simulink model "powerwindow01"  (Simulink 6.0)
settings: Solver=ode23  StartTime=0.0  StopTime=inf  FixedStep=1e-4  RelTol=1e-3
libraries: simulink x4
settings Model: Creator=The MathWorks Inc.  LastModifiedBy=batserve  ExtModeAutoUpdateStatusClock=off
settings DataIOCC: SignalLoggingName=sigsOut
settings OptimizationCC: BooleanDataType=off
settings DebuggingCC: CheckExecutionContextPreStartOutputMsg=on  CheckExecutionContextRuntimeOutputMsg=on  SolverPrmCheckMsg=none
settings HardwareCC: TargetUnknown=on

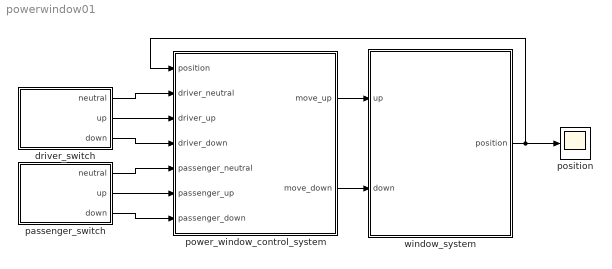
== system powerwindow01 ==
  driver_switch : Subsystem  PropExecContextAcrossSSBoundary=on
  passenger_switch : Subsystem  PropExecContextAcrossSSBoundary=on
  position : Scope
      settings: YMin=-0.05  YMax=0.5  DataFormat=Array
  power_window_control_system : Subsystem  PropExecContextAcrossSSBoundary=on
  window_system : Subsystem  PropExecContextAcrossSSBoundary=on
  wires:
  driver_switch/1(neutral) -> power_window_control_system/2(driver_neutral)
  driver_switch/2(up) -> power_window_control_system/3(driver_up)
  driver_switch/3(down) -> power_window_control_system/4(driver_down)
  passenger_switch/1(neutral) -> power_window_control_system/5(passenger_neutral)
  passenger_switch/2(up) -> power_window_control_system/6(passenger_up)
  passenger_switch/3(down) -> power_window_control_system/7(passenger_down)
  power_window_control_system/1(move_up) -> window_system/1(up)
  power_window_control_system/2(move_down) -> window_system/2(down)
  window_system/1(position) -> position/1, power_window_control_system/1(position)

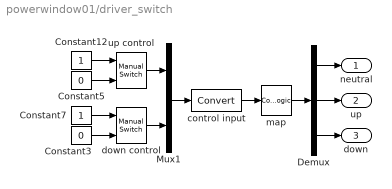
== system powerwindow01/driver_switch ==
  Constant12 : Constant
  Constant3 : Constant  Value=0
  Constant5 : Constant  Value=0
  Constant7 : Constant
  Demux : Demux  Outputs=3
  Mux1 : Mux  Inputs=2
  control input : DataTypeConversion  OutDataTypeMode=boolean  SaturateOnIntegerOverflow=on  RndMeth=Zero
  down control : simulink/Signal Routing/Manual Switch  sw=0  action=0
  map : CombinatorialLogic  TruthTable=[1 0 0;0 0 1;0 1 0;1 0 0]
  up control : simulink/Signal Routing/Manual Switch  sw=0  action=0
  neutral : Outport
  up : Outport  Port=2
  down : Outport  Port=3
  wires:
  control input/1 -> map/1
  Constant12/1 -> up control/1
  Constant5/1 -> up control/2
  Constant7/1 -> down control/1
  Constant3/1 -> down control/2
  down control/1 -> Mux1/2
  Mux1/1 -> control input/1
  up control/1 -> Mux1/1
  map/1 -> Demux/1
  Demux/1 -> neutral/1
  Demux/2 -> up/1
  Demux/3 -> down/1

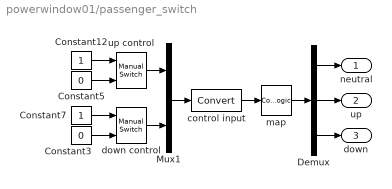
== system powerwindow01/passenger_switch ==
  Constant12 : Constant
  Constant3 : Constant  Value=0
  Constant5 : Constant  Value=0
  Constant7 : Constant
  Demux : Demux  Outputs=3
  Mux1 : Mux  Inputs=2
  control input : DataTypeConversion  OutDataTypeMode=boolean  SaturateOnIntegerOverflow=on  RndMeth=Zero
  down control : simulink/Signal Routing/Manual Switch  sw=0  action=0
  map : CombinatorialLogic  TruthTable=[1 0 0;0 0 1;0 1 0;1 0 0]
  up control : simulink/Signal Routing/Manual Switch  sw=0  action=0
  neutral : Outport
  up : Outport  Port=2
  down : Outport  Port=3
  wires:
  Demux/3 -> down/1
  Demux/2 -> up/1
  Demux/1 -> neutral/1
  map/1 -> Demux/1
  up control/1 -> Mux1/1
  Mux1/1 -> control input/1
  down control/1 -> Mux1/2
  Constant3/1 -> down control/2
  Constant7/1 -> down control/1
  Constant5/1 -> up control/2
  Constant12/1 -> up control/1
  control input/1 -> map/1

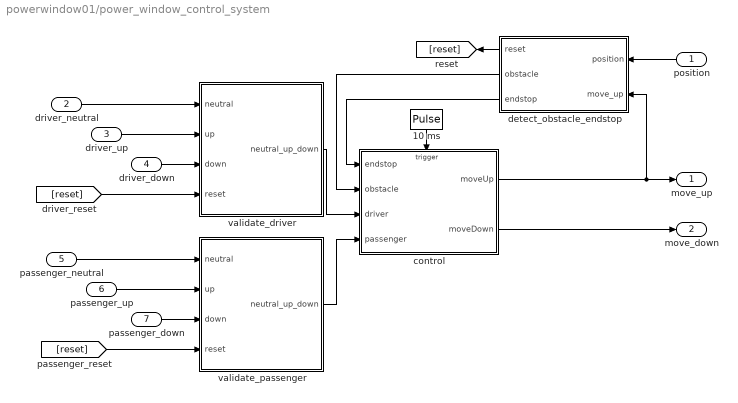
== system powerwindow01/power_window_control_system ==
  position : Inport  Orientation=left  Port=1  LatchInput=off
  driver_neutral : Inport  Port=2  LatchInput=off
  driver_up : Inport  Port=3  LatchInput=off
  driver_down : Inport  Port=4  LatchInput=off
  passenger_neutral : Inport  Port=5  LatchInput=off
  passenger_up : Inport  Port=6  LatchInput=off
  passenger_down : Inport  Port=7  LatchInput=off
  10 ms : DiscretePulseGenerator  Orientation=down  SampleTime=10e-3
  control : Stateflow chart  TreatAsAtomicUnit=on  PropExecContextAcrossSSBoundary=on
  detect_obstacle_endstop : Subsystem  Orientation=left  PropExecContextAcrossSSBoundary=on
  validate_driver : Subsystem  PropExecContextAcrossSSBoundary=on
  validate_passenger : Subsystem  PropExecContextAcrossSSBoundary=on
  move_up : Outport
  move_down : Outport  Port=2
  wires:
  detect_obstacle_endstop/2(obstacle) -> control/2(obstacle)
  detect_obstacle_endstop/3(endstop) -> control/1(endstop)
  detect_obstacle_endstop/1(reset) -> [reset]
  position/1 -> detect_obstacle_endstop/1(position)
  10 ms/1 -> control/Trigger
  control/1(moveUp) -> detect_obstacle_endstop/2(move_up), move_up/1
  control/2(moveDown) -> move_down/1
  driver_neutral/1 -> validate_driver/1(neutral)
  driver_up/1 -> validate_driver/2(up)
  driver_down/1 -> validate_driver/3(down)
  [reset] -> validate_driver/4(reset)
  passenger_neutral/1 -> validate_passenger/1(neutral)
  passenger_up/1 -> validate_passenger/2(up)
  passenger_down/1 -> validate_passenger/3(down)
  [reset] -> validate_passenger/4(reset)
  validate_driver/1(neutral_up_down) -> control/3(driver)
  validate_passenger/1(neutral_up_down) -> control/4(passenger)

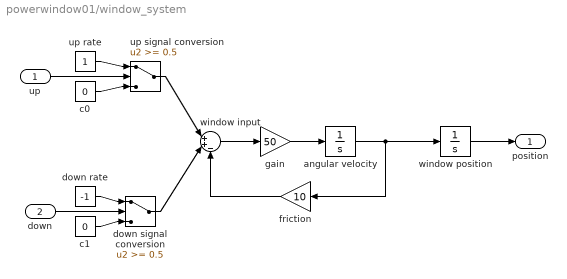
== system powerwindow01/window_system ==
  up : Inport  Port=1  LatchInput=off
  down : Inport  Port=2  LatchInput=off
  angular velocity : Integrator
  c0 : Constant  Value=0
  c1 : Constant  Value=0
  down rate : Constant  Value=-1
  down signal conversion : Switch  Threshold=0.5  InputSameDT=on
  friction : Gain  Orientation=left  Gain=10  SaturateOnIntegerOverflow=on
  gain : Gain  Gain=50  SaturateOnIntegerOverflow=on
  up rate : Constant
  up signal conversion : Switch  Threshold=0.5  InputSameDT=on
  window input : Sum  Inputs=|++-  SaturateOnIntegerOverflow=on  InputSameDT=on
  window position : Integrator
  position : Outport
  wires:
  friction/1 -> window input/3
  angular velocity/1 -> window position/1, friction/1
  gain/1 -> angular velocity/1
  window input/1 -> gain/1
  down signal conversion/1 -> window input/2
  up signal conversion/1 -> window input/1
  c1/1 -> down signal conversion/3
  down rate/1 -> down signal conversion/1
  c0/1 -> up signal conversion/3
  up rate/1 -> up signal conversion/1
  up/1 -> up signal conversion/2
  window position/1 -> position/1
  down/1 -> down signal conversion/2

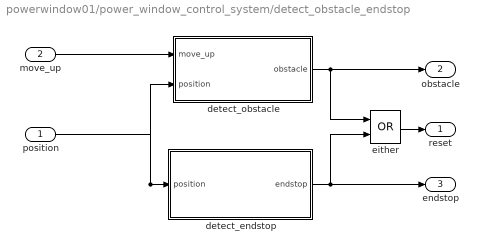
== system powerwindow01/power_window_control_system/detect_obstacle_endstop ==
  position : Inport  Port=1  LatchInput=off
  move_up : Inport  Port=2  LatchInput=off
  detect_endstop : Subsystem  PropExecContextAcrossSSBoundary=on
  detect_obstacle : Subsystem  PropExecContextAcrossSSBoundary=on
  either : Logic  Operator=OR
  reset : Outport
  obstacle : Outport  Port=2
  endstop : Outport  Port=3
  wires:
  detect_obstacle/1(obstacle) -> either/1, obstacle/1
  detect_endstop/1(endstop) -> endstop/1, either/2
  either/1 -> reset/1
  position/1 -> detect_obstacle/2(position), detect_endstop/1(position)
  move_up/1 -> detect_obstacle/1(move_up)

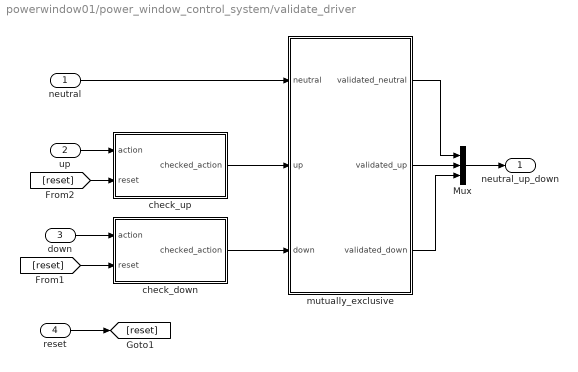
== system powerwindow01/power_window_control_system/validate_driver ==
  neutral : Inport  Port=1  LatchInput=off
  up : Inport  Port=2  LatchInput=off
  down : Inport  Port=3  LatchInput=off
  reset : Inport  Port=4  LatchInput=off
  Mux : Mux  Inputs=3
  check_down : Subsystem  PropExecContextAcrossSSBoundary=on
  check_up : Subsystem  PropExecContextAcrossSSBoundary=on
  mutually_exclusive : Subsystem  PropExecContextAcrossSSBoundary=on
  neutral_up_down : Outport
  wires:
  Mux/1 -> neutral_up_down/1
  reset/1 -> [reset]
  [reset] -> check_down/2(reset)
  [reset] -> check_up/2(reset)
  check_up/1(checked_action) -> mutually_exclusive/2(up)
  neutral/1 -> mutually_exclusive/1(neutral)
  up/1 -> check_up/1(action)
  down/1 -> check_down/1(action)
  mutually_exclusive/1(validated_neutral) -> Mux/1
  mutually_exclusive/2(validated_up) -> Mux/2
  mutually_exclusive/3(validated_down) -> Mux/3
  check_down/1(checked_action) -> mutually_exclusive/3(down)

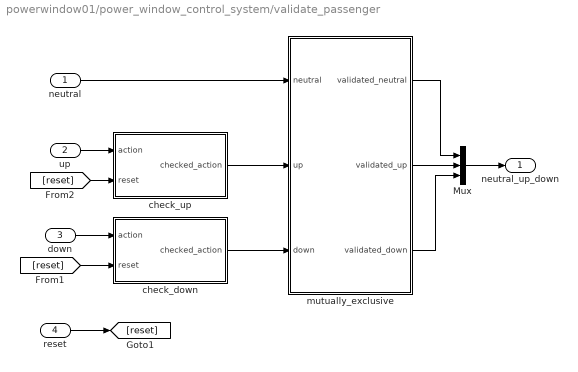
== system powerwindow01/power_window_control_system/validate_passenger ==
  neutral : Inport  Port=1  LatchInput=off
  up : Inport  Port=2  LatchInput=off
  down : Inport  Port=3  LatchInput=off
  reset : Inport  Port=4  LatchInput=off
  Mux : Mux  Inputs=3
  check_down : Subsystem  PropExecContextAcrossSSBoundary=on
  check_up : Subsystem  PropExecContextAcrossSSBoundary=on
  mutually_exclusive : Subsystem  PropExecContextAcrossSSBoundary=on
  neutral_up_down : Outport
  wires:
  Mux/1 -> neutral_up_down/1
  reset/1 -> [reset]
  [reset] -> check_down/2(reset)
  [reset] -> check_up/2(reset)
  check_up/1(checked_action) -> mutually_exclusive/2(up)
  neutral/1 -> mutually_exclusive/1(neutral)
  up/1 -> check_up/1(action)
  down/1 -> check_down/1(action)
  mutually_exclusive/1(validated_neutral) -> Mux/1
  mutually_exclusive/2(validated_up) -> Mux/2
  mutually_exclusive/3(validated_down) -> Mux/3
  check_down/1(checked_action) -> mutually_exclusive/3(down)

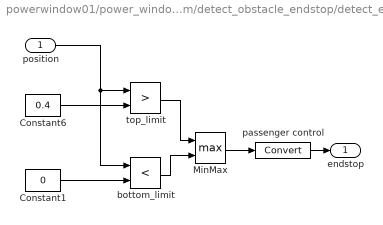
== system powerwindow01/power_window_control_system/detect_obstacle_endstop/detect_endstop ==
  position : Inport  Port=1  LatchInput=off
  Constant1 : Constant  Value=0
  Constant6 : Constant  Value=0.4
  MinMax : MinMax  Function=max  Inputs=2  SaturateOnIntegerOverflow=on  InputSameDT=on
  bottom_limit : RelationalOperator  Operator=<  InputSameDT=on
  passenger control : DataTypeConversion  OutDataTypeMode=boolean  SaturateOnIntegerOverflow=on  RndMeth=Zero
  top_limit : RelationalOperator  Operator=>  InputSameDT=on
  endstop : Outport
  wires:
  passenger control/1 -> endstop/1
  position/1 -> top_limit/1, bottom_limit/1
  Constant6/1 -> top_limit/2
  Constant1/1 -> bottom_limit/2
  MinMax/1 -> passenger control/1
  top_limit/1 -> MinMax/1
  bottom_limit/1 -> MinMax/2

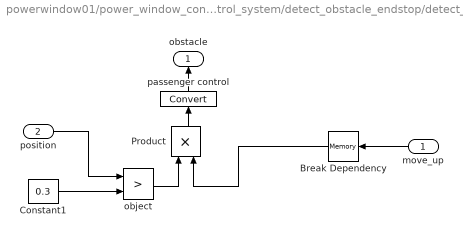
== system powerwindow01/power_window_control_system/detect_obstacle_endstop/detect_obstacle ==
  move_up : Inport  Orientation=left  Port=1  LatchInput=off
  position : Inport  Port=2  LatchInput=off
  Break Dependency : Memory  Orientation=left
  Constant1 : Constant  Value=0.3
  Product : Product  Orientation=up  SaturateOnIntegerOverflow=on  InputSameDT=on
  object : RelationalOperator  Operator=>  InputSameDT=on
  passenger control : DataTypeConversion  Orientation=up  OutDataTypeMode=boolean  SaturateOnIntegerOverflow=on  RndMeth=Zero
  obstacle : Outport  Orientation=up
  wires:
  passenger control/1 -> obstacle/1
  Product/1 -> passenger control/1
  Break Dependency/1 -> Product/2
  move_up/1 -> Break Dependency/1
  position/1 -> object/1
  object/1 -> Product/1
  Constant1/1 -> object/2

== system powerwindow01/power_window_control_system/validate_driver/check_down ==
  action : Inport  Port=1  LatchInput=off
  reset : Inport  Port=2  LatchInput=off
  allow_action : Logic
  overrule : Logic  Operator=NOT
  checked_action : Outport
  wires:
  reset/1 -> overrule/1
  allow_action/1 -> checked_action/1
  action/1 -> allow_action/1
  overrule/1 -> allow_action/2

== system powerwindow01/power_window_control_system/validate_driver/check_up ==
  action : Inport  Port=1  LatchInput=off
  reset : Inport  Port=2  LatchInput=off
  allow_action : Logic
  overrule : Logic  Operator=NOT
  checked_action : Outport
  wires:
  overrule/1 -> allow_action/2
  action/1 -> allow_action/1
  allow_action/1 -> checked_action/1
  reset/1 -> overrule/1

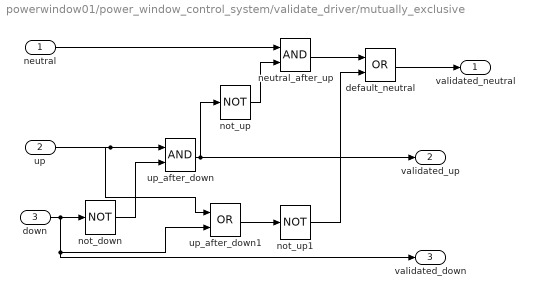
== system powerwindow01/power_window_control_system/validate_driver/mutually_exclusive ==
  neutral : Inport  Port=1  LatchInput=off
  up : Inport  Port=2  LatchInput=off
  down : Inport  Port=3  LatchInput=off
  default_neutral : Logic  Operator=OR
  neutral_after_up : Logic
  not_down : Logic  Operator=NOT
  not_up : Logic  Operator=NOT
  not_up1 : Logic  Operator=NOT
  up_after_down : Logic
  up_after_down1 : Logic  Operator=OR
  validated_neutral : Outport
  validated_up : Outport  Port=2
  validated_down : Outport  Port=3
  wires:
  not_down/1 -> up_after_down/2
  up_after_down/1 -> not_up/1, validated_up/1
  not_up/1 -> neutral_after_up/2
  down/1 -> not_down/1, up_after_down1/2, validated_down/1
  neutral/1 -> neutral_after_up/1
  up/1 -> up_after_down/1, up_after_down1/1
  up_after_down1/1 -> not_up1/1
  neutral_after_up/1 -> default_neutral/1
  default_neutral/1 -> validated_neutral/1
  not_up1/1 -> default_neutral/2

== system powerwindow01/power_window_control_system/validate_passenger/check_down ==
  action : Inport  Port=1  LatchInput=off
  reset : Inport  Port=2  LatchInput=off
  allow_action : Logic
  overrule : Logic  Operator=NOT
  checked_action : Outport
  wires:
  reset/1 -> overrule/1
  allow_action/1 -> checked_action/1
  action/1 -> allow_action/1
  overrule/1 -> allow_action/2

== system powerwindow01/power_window_control_system/validate_passenger/check_up ==
  action : Inport  Port=1  LatchInput=off
  reset : Inport  Port=2  LatchInput=off
  allow_action : Logic
  overrule : Logic  Operator=NOT
  checked_action : Outport
  wires:
  overrule/1 -> allow_action/2
  action/1 -> allow_action/1
  allow_action/1 -> checked_action/1
  reset/1 -> overrule/1

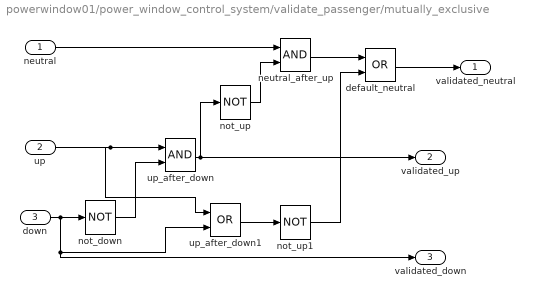
== system powerwindow01/power_window_control_system/validate_passenger/mutually_exclusive ==
  neutral : Inport  Port=1  LatchInput=off
  up : Inport  Port=2  LatchInput=off
  down : Inport  Port=3  LatchInput=off
  default_neutral : Logic  Operator=OR
  neutral_after_up : Logic
  not_down : Logic  Operator=NOT
  not_up : Logic  Operator=NOT
  not_up1 : Logic  Operator=NOT
  up_after_down : Logic
  up_after_down1 : Logic  Operator=OR
  validated_neutral : Outport
  validated_up : Outport  Port=2
  validated_down : Outport  Port=3
  wires:
  not_down/1 -> up_after_down/2
  up_after_down/1 -> not_up/1, validated_up/1
  not_up/1 -> neutral_after_up/2
  down/1 -> not_down/1, up_after_down1/2, validated_down/1
  neutral/1 -> neutral_after_up/1
  up/1 -> up_after_down/1, up_after_down1/1
  up_after_down1/1 -> not_up1/1
  neutral_after_up/1 -> default_neutral/1
  default_neutral/1 -> validated_neutral/1
  not_up1/1 -> default_neutral/2

== stateflow chart power_window_control_system/control ==
  settings: executeAtInitialization=1
  state emergencyDown
    entry:
    moveUp = 0;
    moveDown = 1;
  state safe
    state driverUp
      entry: moveUp = 1;
      exit: moveUp = 0;
      state iniDriverUp
      state DriverUp
      state autoDriverUp
      iniDriverUp -> (junction 26) : after(100,ticks)
      (junction 26) -> DriverUp
      (junction 26) -> autoDriverUp : [driver[1]]
    state driverDown
      entry: moveDown = 1;
      exit: moveDown = 0;
      state iniDriverDown
      state DriverDown
      state autoDriverDown
      iniDriverDown -> (junction 25) : after(100,ticks)
      (junction 25) -> autoDriverDown : [driver[1]]
      (junction 25) -> DriverDown
    state driverNeutral
      entry:
      moveUp = 0;
      moveDown = 0;
      state passengerneutral
        entry:
        moveUp = 0;
        moveDown = 0;
      state passengerUp
        entry: moveUp = 1;
        exit: moveUp = 0;
        state iniPassengerUp
        state PassengerUp
        state autoPassengerUp
        (junction 24) -> PassengerUp
        (junction 24) -> autoPassengerUp : [passenger[1]]
        iniPassengerUp -> (junction 24) : after(100,ticks)
      state passengerDown
        entry: moveDown = 1;
        exit: moveDown = 0;
        state iniPassengerDown
        state passengerDown
        state autoPassengerDown
        (junction 23) -> autoPassengerDown : [passenger[1]]
        iniPassengerDown -> (junction 23) : after(100,ticks)
        (junction 23) -> safe.driverNeutral.passengerDown.passengerDown
      safe.driverNeutral.passengerDown.passengerDown -> passengerneutral : [passenger[1]]
      safe.driverNeutral.passengerDown -> passengerneutral : [endstop]
      PassengerUp -> passengerneutral : [passenger[1]]
      passengerUp -> passengerneutral : [endstop]
      passengerneutral -> iniPassengerDown : [passenger[3]]
      passengerneutral -> iniPassengerUp : [passenger[2]]
      safe.driverNeutral.passengerDown -> PassengerUp : [passenger[2]]
      passengerUp -> safe.driverNeutral.passengerDown.passengerDown : [passenger[3]]
      (default) -> passengerneutral
    driverNeutral -> iniDriverDown : [driver[3]]
    driverUp -> DriverDown : [driver[3]]
    driverDown -> DriverUp : [driver[2]]
    driverNeutral -> iniDriverUp : [driver[2]]
    DriverDown -> driverNeutral : [driver[1]]
    DriverUp -> driverNeutral : [driver[1]]
    driverDown -> driverNeutral : [endstop]
    driverUp -> driverNeutral : [endstop]
    (default) -> driverNeutral
  emergencyDown -> passengerneutral : [endstop | after(100,ticks)]
  safe -> emergencyDown : [obstacle]
  (default) -> safe
  data: moveUp output double; moveDown output double; endstop input boolean; obstacle input boolean; driver input boolean size=3; passenger input boolean size=3
  events: ticks input EITHER_EDGE_EVENT
